simulink model "SISO_Sim_b2"  (R2015b)
settings: Solver=VariableStepAuto  StartTime=0.0  StopTime=15  RelTol=1e-3
libraries: simulink_extras x4, simulink x1
settings Model: Creator=dmartin_a  LastModifiedBy=dmartin_a

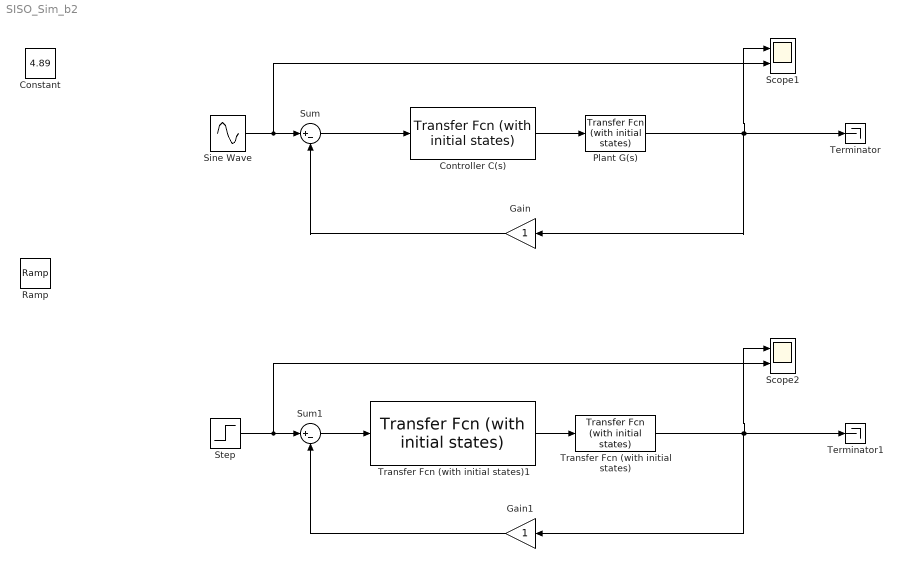
== system SISO_Sim_b2 ==
  Constant : Constant  Value=4.89  SampleTime=.01
  Controller C(s) : simulink_extras/Additional Linear/Transfer Fcn (with initial states)  N=[1 -10996.8 -395573]  D=[1 2792 1]  X0=0
  Gain : Gain
  Gain1 : Gain
  Plant G(s) : simulink_extras/Additional Linear/Transfer Fcn (with initial states)  N=[-316]  D="[1  -976]"  X0=0
  Ramp : simulink/Sources/Ramp  slope=2  start=5  X0=0
  Scope1 : Scope  NumInputPorts=2
  Scope2 : Scope  NumInputPorts=2
  Sine Wave : Sin  Amplitude=200  Frequency=20  Phase=1  SampleTime=0
  Step : Step  Time=5  SampleTime=0
  Sum : Sum  Inputs=|+-
  Sum1 : Sum  Inputs=|+-
  Terminator : Terminator
  Terminator1 : Terminator
  Transfer Fcn (with initial states) : simulink_extras/Additional Linear/Transfer Fcn (with initial states)  N=[31.62 -0.1]  D="[1  -24.4 0 0]"  X0=2
  Transfer Fcn (with initial states)1 : simulink_extras/Additional Linear/Transfer Fcn (with initial states)  N=[1 1 3.248e12 -3.1625e13 -1e11]  D=[1 1 1000 524.3984 -1.02e14]  X0=1
  wires:
  Controller C(s)/1 -> Plant G(s)/1
  Sum/1 -> Controller C(s)/1
  Plant G(s)/1 -> Terminator/1, Scope1/1, Gain/1
  Gain/1 -> Sum/2
  Sine Wave/1 -> Scope1/2, Sum/1
  Transfer Fcn (with initial states)/1 -> Gain1/1, Scope2/1, Terminator1/1
  Gain1/1 -> Sum1/2
  Step/1 -> Sum1/1, Scope2/2
  Sum1/1 -> Transfer Fcn (with initial states)1/1
  Transfer Fcn (with initial states)1/1 -> Transfer Fcn (with initial states)/1
